simulink model "ABB_1010"  (R2024a)
settings: Solver=VariableStepAuto  StartTime=0.0  StopTime=200  RelTol=1e-3
model workspace: external: MATLAB File C:\Users\lucas\OneDrive\Documents\MATLAB\projeto final\ABB_1010_DataFile.m (data not in the file)
values from neighbouring files (symbols this model uses):
  g = 9.81    [inicializacaoAntropomorfico.m]
  I1 = [ 0.00243841  0.00000307  0.00007261    [inicializacaoAntropomorfico.m]
  I2 = [ 0.01633569  0.00000387 -0.00034405    [inicializacaoAntropomorfico.m]
  I3 = [ 0.00244760 -0.00000208  0.00000538    [inicializacaoAntropomorfico.m]
  I4 = [ 0.00245792 -0.00000008  0.00003121    [inicializacaoAntropomorfico.m]
  I5 = [ 0.00062165 -0.00000206 -0.00000303    [inicializacaoAntropomorfico.m]
  I6 = [ 0.00000357  0.00000000  0.00000000    [inicializacaoAntropomorfico.m]
  I7 = [(m7*L7^2)/12 0.00000000  0.00000000    [inicializacaoAntropomorfico.m]
  L = [L1, L2, L3, L4, L5, L6, L7]    [inicializacaoAntropomorfico.m]
  Lcm1 = [-0.00258308  0.00024508 -0.01434968]    [inicializacaoAntropomorfico.m]
  Lcm2 = [-0.02078894  0.00020016 -0.10516734]    [inicializacaoAntropomorfico.m]
  Lcm3 = [ 0.00021912  0.00015355 -0.06228290]    [inicializacaoAntropomorfico.m]
  Lcm4 = [-0.00172658 -0.00124140 -0.07369196]    [inicializacaoAntropomorfico.m]
  Lcm5 = [-0.00014110  0.00085992 -0.03825278]    [inicializacaoAntropomorfico.m]
  Lcm6 = [ 0.00002478  0.00000000 -0.00042157]    [inicializacaoAntropomorfico.m]
  Lcm7 = [ 0           0          -0.05000000]    [inicializacaoAntropomorfico.m]
  m = [m1, m2, m3, m4, m5, m6, m7]    [inicializacaoAntropomorfico.m]
  Pf = [  0.05    [inicializacaoAntropomorfico.m]
  Pi = [  0.2    [inicializacaoAntropomorfico.m]
  Raio = [0]    [inicializacaoAntropomorfico.m]
  Sentido = [0]    [inicializacaoAntropomorfico.m]
  Tipo = [1]    [inicializacaoAntropomorfico.m]
undefined symbols (not defined in the file or in its folder): smiData, X, Y, Z
libraries: sm_lib x35, nesl_utility x7
(part 13 of 16)

== matlab function ABB_1010/Controle ==
  data: M input; Tc output; H input; G input; C input; Qd input; dQd input; d2Qd input; Q input; dQ input; kp parameter
function Tc = Controlador(M, H, G, C, Qd, dQd, d2Qd, Q, dQ, kp)

    g  = 9.81;
    KP = kp * eye(6);            % Ganho proporcional
    KD = 2 * sqrt(kp) * eye(6);  % Ganho derivativo
    erro = Qd - Q;
    erro_dot = dQd - dQ;
    Tc = M * (d2Qd + KD * erro_dot + KP * erro) + H + C + G;

== matlab function ABB_1010/Plant ==
  data: M input; H input; G input; C input; Tc input; d2Q output
function d2Q  = planta(M,H,G,C,Tc)
    d2Q = zeros(6,1);
    d2Q = M\(Tc-H-C-G);
end

== matlab function ABB_1010/Dinamica1/MATLAB Function2 ==
  data: G output; I1 parameter; L parameter; Lcm1 parameter; Q input; I2 parameter; I3 parameter; I4 parameter; I5 parameter; I6 parameter; Lcm2 parameter; Lcm3 parameter; Lcm4 parameter; Lcm5 parameter; Lcm6 parameter; g parameter; m parameter; I7 parameter; Lcm7 parameter
function G = func_G(I1, L, Lcm1, Q, I2, I3, I4, I5, I6, Lcm2, Lcm3, Lcm4, Lcm5, Lcm6, g, m, I7, Lcm7)
%func_G
%    OUT1 = func_G(Lx2,Lx3,Lxcm2,Lxcm3,Lxcm4,Lxcm5,Lxcm6,Lycm4,Lycm5,Lycm6,Lz4,Lz5,Lzcm2,Lzcm3,Lzcm4,Lzcm5,Lzcm6,Q2,Q3,Q4,Q5,Q6,g,g,g,g,g,M2,M3,M4,M5,M6)

%    This function was generated by the Symbolic Math Toolbox version 24.1.
%    30-Apr-2025 06:22:17
G   = zeros(6,1);
m1  = m(1);
m2  = m(2);
m3  = m(3);
m4  = m(4);
m5  = m(5);
m6  = m(6);
m7  = m(7);

Q1  = Q(1);
Q2  = Q(2);
Q3  = Q(3);
Q4  = Q(4);
Q5  = Q(5);
Q6  = Q(6);

Lz1 = L(1);
Lx2 = L(2);
Lx3 = L(3);
Lx4 = L(4);
Lz5 = L(5);
Lz6 = L(6);
Lz7 = L(7);

Lxcm1 = Lcm1(1);
Lycm1 = Lcm1(2);
Lzcm1 = Lcm1(3);

Lxcm2 = Lcm2(1);
Lycm2 = Lcm2(2);
Lzcm2 = Lcm2(3);

Lxcm3 = Lcm3(1);
Lycm3 = Lcm3(2);
Lzcm3 = Lcm3(3);

Lxcm4 = Lcm4(1);
Lycm4 = Lcm4(2);
Lzcm4 = Lcm4(3);

Lxcm5 = Lcm5(1);
Lycm5 = Lcm5(2);
Lzcm5 = Lcm5(3);

Lxcm6 = Lcm6(1);
Lycm6 = Lcm6(2);
Lzcm6 = Lcm6(3);

Lxcm7 = Lcm7(1);
Lycm7 = Lcm7(2);
Lzcm7 = Lcm7(3);

Ixx1 = I1(1,1);
Ixy1 = I1(1,2);
Ixz1 = I1(1,3);
Iyx1 = I1(2,1);
Iyy1 = I1(2,2);
Iyz1 = I1(2,3);
Izx1 = I1(3,1);
Izy1 = I1(3,2);
Izz1 = I1(3,3);

Ixx2 = I2(1,1);
Ixy2 = I2(1,2);
Ixz2 = I2(1,3);
Iyx2 = I2(2,1);
Iyy2 = I2(2,2);
Iyz2 = I2(2,3);
Izx2 = I2(3,1);
Izy2 = I2(3,2);
Izz2 = I2(3,3);

Ixx3 = I3(1,1);
Ixy3 = I3(1,2);
Ixz3 = I3(1,3);
Iyx3 = I3(2,1);
Iyy3 = I3(2,2);
Iyz3 = I3(2,3);
Izx3 = I3(3,1);
Izy3 = I3(3,2);
Izz3 = I3(3,3);

Ixx4 = I4(1,1);
Ixy4 = I4(1,2);
Ixz4 = I4(1,3);
Iyx4 = I4(2,1);
Iyy4 = I4(2,2);
Iyz4 = I4(2,3);
Izx4 = I4(3,1);
Izy4 = I4(3,2);
Izz4 = I4(3,3);

Ixx5 = I5(1,1);
Ixy5 = I5(1,2);
Ixz5 = I5(1,3);
Iyx5 = I5(2,1);
Iyy5 = I5(2,2);
Iyz5 = I5(2,3);
Izx5 = I5(3,1);
Izy5 = I5(3,2);
Izz5 = I5(3,3);

Ixx6 = I6(1,1);
Ixy6 = I6(1,2);
Ixz6 = I6(1,3);
Iyx6 = I6(2,1);
Iyy6 = I6(2,2);
Iyz6 = I6(2,3);
Izx6 = I6(3,1);
Izy6 = I6(3,2);
Izz6 = I6(3,3);

Ixx7 = I7(1,1);
Ixy7 = I7(1,2);
Ixz7 = I7(1,3);
Iyx7 = I7(2,1);
Iyy7 = I7(2,2);
Iyz7 = I7(2,3);
Izx7 = I7(3,1);
Izy7 = I7(3,2);
Izz7 = I7(3,3);

t2 = cos(Q2);
t3 = cos(Q4);
t4 = cos(Q5);
t5 = cos(Q6);
t6 = sin(Q4);
t7 = sin(Q5);
t8 = sin(Q6);
t9 = Q2+Q3;
t10 = Q4+Q5;
t13 = -Q5;
t11 = cos(t9);
t12 = sin(t9);
t14 = Q4+t13;
t15 = Lx3*g*m3*t11;
t16 = Lx3*g*m4*t11;
t17 = Lx3*g*m5*t11;
t18 = Lx3*g*m6*t11;
t19 = Lxcm3*g*m3*t11;
t20 = Lzcm3*g*m3*t12;
t21 = Lzcm4*g*m4*t12;
t22 = Lx4*g*m4*t3*t11;
t23 = Lx4*g*m5*t3*t11;
t24 = Lx4*g*m6*t3*t11;
t25 = Lxcm4*g*m4*t3*t11;
t26 = Lycm4*g*m4*t6*t11;
t27 = Lycm5*g*m5*t6*t11;
t28 = Lz6*g*m6*t4*t12;
t29 = Lzcm5*g*m5*t4*t12;
t30 = Lzcm6*g*m6*t4*t12;
t31 = Lxcm5*g*m5*t7*t12;
t39 = Lycm6*g*m6*t5*t6*t11;
t40 = Lz6*g*m6*t3*t7*t11;
t41 = Lzcm6*g*m6*t3*t7*t11;
t42 = Lxcm6*g*m6*t6*t8*t11;
t43 = Lxcm6*g*m6*t5*t7*t12;
t44 = Lycm6*g*m6*t7*t8*t12;
t52 = Lxcm6*g*m6*t3*t4*t5*t11;
t53 = Lycm6*g*m6*t3*t4*t8*t11;
t32 = -t15;
t33 = -t16;
t34 = -t17;
t35 = -t18;
t36 = -t19;
t37 = -t20;
t38 = -t21;
t45 = -t22;
t46 = -t23;
t47 = -t24;
t48 = -t25;
t49 = -t28;
t50 = -t29;
t51 = -t30;
t54 = -t40;
t55 = -t41;
t56 = -t44;
t57 = -t52;
mt1 = [0.0;t26+t27+t31+t32+t33+t34+t35+t36+t37+t38+t39+t42+t43+t45+t46+t47+t48+t49+t50+t51+t53+t54+t55+t56+t57-Lzcm2*g*m2*sin(Q2)-Lx2*g*m2*t2-Lx2*g*m3*t2-Lx2*g*m4*t2-Lx2*g*m5*t2-Lx2*g*m6*t2-Lxcm2*g*m2*t2-(Lxcm5*g*m5*t11*cos(t10))./2.0-(Lxcm5*g*m5*t11*cos(t14))./2.0-(Lzcm5*g*m5*t11*sin(t10))./2.0+(Lzcm5*g*m5*t11*sin(t14))./2.0;t26+t27+t31+t32+t33+t34+t35+t36+t37+t38+t39+t42+t43+t45+t46+t47+t48+t49+t50+t51+t53+t54+t55+t56+t57-Lxcm5*g*m5*t3*t4*t11-Lzcm5*g*m5*t3*t7*t11];
mt2 = [t12*(Lx4*g*m4*t6+Lx4*g*m5*t6+Lx4*g*m6*t6+Lxcm4*g*m4*t6+Lycm4*g*m4*t3+Lycm5*g*m5*t3+Lxcm5*g*m5*t4*t6+Lxcm6*g*m6*t3*t8+Lycm6*g*m6*t3*t5+Lz6*g*m6*t6*t7+Lzcm5*g*m5*t6*t7+Lzcm6*g*m6*t6*t7+Lxcm6*g*m6*t4*t5*t6-Lycm6*g*m6*t4*t6*t8);t3*t31+t3*t43+t3*t49+t3*t50+t3*t51+t3*t56-Lxcm5*g*m5*t4*t11-Lz6*g*m6*t7*t11-Lzcm5*g*m5*t7*t11-Lzcm6*g*m6*t7*t11-Lxcm6*g*m6*t4*t5*t11+Lycm6*g*m6*t4*t8*t11;g*m6*(Lxcm6*t5*t6*t12+Lxcm6*t7*t8*t11+Lycm6*t5*t7*t11-Lycm6*t6*t8*t12+Lxcm6*t3*t4*t8*t12+Lycm6*t3*t4*t5*t12)];
out1 = [mt1;mt2];
end
